simulink model "modelCopy"  (R2018b)
settings: Solver=VariableStepAuto  StartTime=0.0  StopTime=50  RelTol=1e-3
libraries: simulink x1, powerlib_meascontrol x1
settings Model: Creator=computer  LastModifiedBy=computer

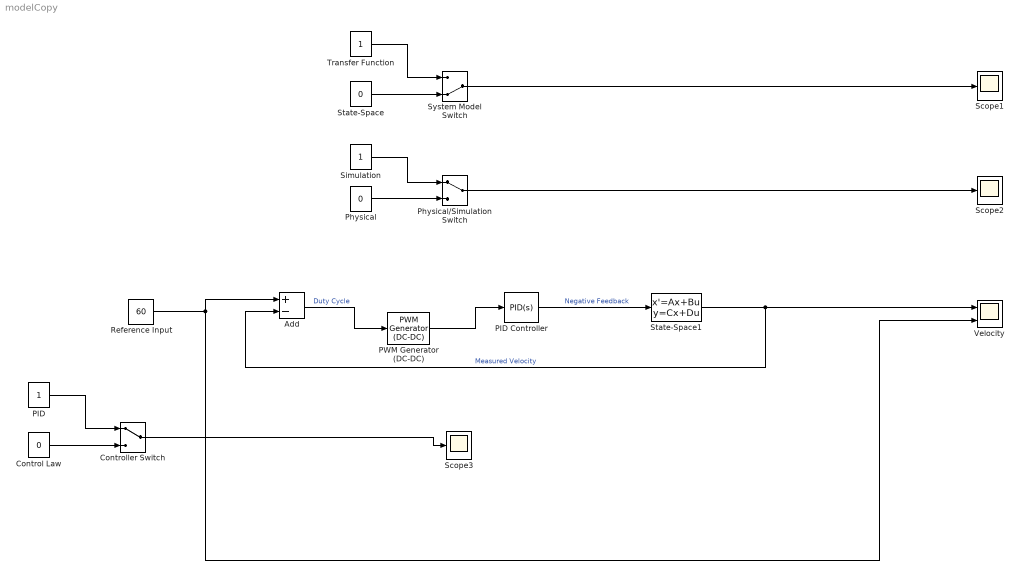
== system modelCopy ==
  Add : Sum  Inputs=+-
  Control Law : Constant  Value=0
  Controller Switch : ManualSwitch
  PID : Constant
  PID Controller : simulink/Continuous/PID Controller  Controller=PID  Form=Parallel  TimeDomain=Continuous-time  SampleTime=-1  IntegratorMethod=Forward Euler  FilterMethod=Forward Euler  ControllerParametersSource=internal  P=10  I=10  D=0  UseFilter=on  N=100  TunerSelectOption=Transfer Function Based (PID Tuner App)  InitialConditionSource=internal  InitialConditionForIntegrator=0  InitialConditionForFilter=0  DifferentiatorICPrevScaledInput=0  ExternalReset=none  TrackingMode=off  Kt=1  LimitOutput=off  UpperSaturationLimit=inf  LowerSaturationLimit=-inf  LinearizeAsGain=on  AntiWindupMode=none  Kb=1  POutMin=[]  POutMax=[]  IOutMin=[]  IOutMax=[]  DOutMin=[]  DOutMax=[]  NOutMin=[]  NOutMax=[]  SumOutMin=[]  SumOutMax=[]  SaturationOutMin=[]  SaturationOutMax=[]  PParamMin=[]  PParamMax=[]  IParamMin=[]  IParamMax=[]  DParamMin=[]  DParamMax=[]  NParamMin=[]  NParamMax=[]  KbParamMin=[]  KbParamMax=[]  KtParamMin=[]  KtParamMax=[]  KbOutMin=[]  KbOutMax=[]  KtOutMin=[]  KtOutMax=[]  IntegratorOutMin=[]  IntegratorOutMax=[]  FilterOutMin=[]  FilterOutMax=[]  SumI1OutMin=[]  SumI1OutMax=[]  SumI2OutMin=[]  SumI2OutMax=[]  SumI3OutMin=[]  SumI3OutMax=[]  SumI4OutMin=[]  SumI4OutMax=[]  SumDOutMin=[]  SumDOutMax=[]  DifferentiatorOutMin=[]  DifferentiatorOutMax=[]  FilterDiffOutCoefMin=[]  FilterDiffOutCoefMax=[]  ReciprocalOutMin=[]  ReciprocalOutMax=[]  SumDenOutMin=[]  SumDenOutMax=[]  SumNumOutMin=[]  SumNumOutMax=[]  DivideOutMin=[]  DivideOutMax=[]  IntegratorContinuousStateAttributes=''  IntegratorStateMustResolveToSignalObject=off  IntegratorRTWStateStorageClass=Auto  FilterContinuousStateAttributes=''  FilterStateMustResolveToSignalObject=off  FilterRTWStateStorageClass=Auto  ParallelPVariant=InternalParameters  IdealPVariant=Disabled  IVariant=InternalParameters  DVariant=InternalParameters  IntegratorVariant=Continuous  SatVariant=Disabled  AWVariant=Passthrough  PCopyVariant=Disabled  TRVariant=Disabled  FdbkBlocksVariant=Forward  IdealPFdbkVariant=Disabled  SatFdbkVariant=Disabled  DerivativeFilterVariant=ContFilter  NVariant=InternalParameters  NCopyVariant=Disabled  FilterICVariant=InternalICsFilter  IntegratorICVariant=InternalICs  ExternalResetVariant=Disabled  TRSumVariant=Passthrough  SumFdbkVariant=Disabled  SumVariant=Sum_PID
  PWM Generator (DC-DC) : powerlib_meascontrol/Pulse & Signal Generators/PWM Generator (DC-DC)  Fsw=5000  Ts=.0001
  Physical : Constant  Value=0
  Physical/Simulation Switch : ManualSwitch
  Reference Input : Constant  Value=60
  Scope1 : Scope
  Scope2 : Scope
  Scope3 : Scope
  "Simulation " : Constant
  State-Space : Constant  Value=0
  State-Space1 : StateSpace  D=0  InitialCondition=0
  System Model Switch : ManualSwitch  CurrentSetting=0
  Transfer Function : Constant
  Velocity : Scope  NumInputPorts=2
  wires:
  Physical/1 -> Physical/Simulation Switch/2
  "Simulation "/1 -> Physical/Simulation Switch/1
  Control Law/1 -> Controller Switch/2
  PID/1 -> Controller Switch/1
  State-Space/1 -> System Model Switch/2
  Transfer Function/1 -> System Model Switch/1
  Reference Input/1 -> Velocity/2, Add/1
  Add/1 -> PWM Generator (DC-DC)/1  "Duty Cycle"
  Physical/Simulation Switch/1 -> Scope2/1
  System Model Switch/1 -> Scope1/1
  State-Space1/1 -> Add/2, Velocity/1  "Measured Velocity"
  Controller Switch/1 -> Scope3/1
  PID Controller/1 -> State-Space1/1  "Negative Feedback"
  PWM Generator (DC-DC)/1 -> PID Controller/1
